simulink model "scMobileRobotLogicalArchitecture_Initial"  (R2022a)
settings: Solver=VariableStepAuto  StartTime=0.0  StopTime=10.0  RelTol=1e-3
model workspace (MAT data in the model file):
  CameraInterface = Simulink.Bus
  CameraInterface.Alignment = -1
  CameraInterface.PreserveElementDimensions = 0
  CameraInterface.Elements_internal(1) = Simulink.BusElement
  CameraInterface.Elements_internal(1).DimensionsMode = 'Fixed'
  CameraInterface.Elements_internal(1).SamplingMode = 'Sample based'
  CameraInterface.Elements_internal(1).SampleTime = -1
  CameraInterface.Elements_internal(1).Name = 'imageData'
  CameraInterface.Elements_internal(1).DataType_internal = 'uint16'
  CameraInterface.Elements_internal(1).Complexity = 'real'
  CameraInterface.Elements_internal(1).Dimensions = 1
  CameraInterface.Elements_internal(2) = Simulink.BusElement
  CameraInterface.Elements_internal(2).DimensionsMode = 'Fixed'
  CameraInterface.Elements_internal(2).SamplingMode = 'Sample based'
  CameraInterface.Elements_internal(2).SampleTime = -1
  CameraInterface.Elements_internal(2).Name = 'geoLoc'
  CameraInterface.Elements_internal(2).DataType_internal = 'double'
  CameraInterface.Elements_internal(2).Complexity = 'real'
  CameraInterface.Elements_internal(2).Dimensions = 1
  CameraInterface.Elements_internal(3) = Simulink.BusElement
  CameraInterface.Elements_internal(3).DimensionsMode = 'Fixed'
  CameraInterface.Elements_internal(3).SamplingMode = 'Sample based'
  CameraInterface.Elements_internal(3).SampleTime = -1
  CameraInterface.Elements_internal(3).Name = 'healthCheck'
  CameraInterface.Elements_internal(3).DataType_internal = 'int8'
  CameraInterface.Elements_internal(3).Complexity = 'real'
  CameraInterface.Elements_internal(3).Dimensions = 1
  CameraInterface.DataScope = 'Auto'
  CommandType = Simulink.ValueType
  CommandType.DataType = 'Enum: CommandEnum'
  GroundInterface = Simulink.ConnectionBus
  GroundInterface.Elements_internal(1) = Simulink.ConnectionElement
  GroundInterface.Elements_internal(1).Name = 'fixture'
  GroundInterface.Elements_internal(1).Type_internal = 'foundation.mechanical.translational.translational'
  GroundInterface.Elements_internal(2) = Simulink.ConnectionElement
  GroundInterface.Elements_internal(2).Name = 'socket'
  GroundInterface.Elements_internal(2).Type_internal = 'foundation.mechanical.rotational.rotational'
settings Model: Creator=The MathWorks, Inc.  LastModifiedBy=The MathWorks, Inc.
settings SolverCC: AlgebraicLoopSolver=TrustRegion  AutoInsertRateTranBlk=on  MaxZcPerStep=1
settings DebuggingCC: UnconnectedInputMsg=warning  UnconnectedOutputMsg=warning  UnconnectedLineMsg=warning  SFMachineParentedDataDiag=warning
settings ModelReferenceCC: ModelReferenceNumInstancesAllowed=Single
settings RTWCC: DLArmComputeVersion=19.05

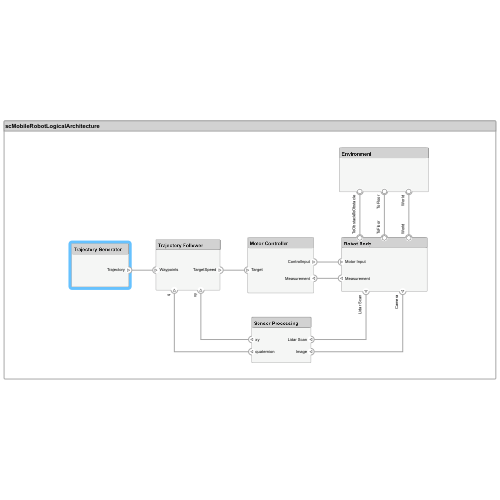
[thumbnail: Simulink's stored preview of the top-level diagram]
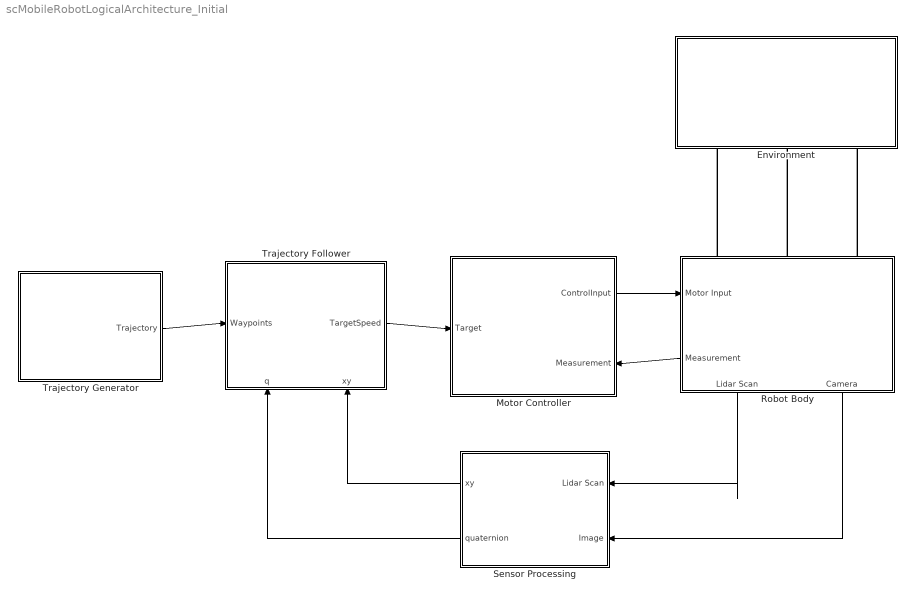
== system scMobileRobotLogicalArchitecture_Initial ==
  Environment : Subsystem
      settings: PortSchema="{\"entries\":[{\"content\":{\"headerSize\":26,\"margin\":15,\"minimumSpacing\":25,\"sides\":[{\"content\":{\"connectorIds\":[]},\"type\":\"ConnectorPlacement.EquallySpacedRectSide\",\"uuid\":\"636813ac-2488-43df-bc25-3d2ab9c69d6b\"},{\"content\":{\"connectorIds\":[],\"side\":\"RIGHT\"},\"type\":\"ConnectorPlacement.EquallySpacedRectSide\",\"uuid\":\"1c2f400a-ff06-4f0e-a520-9265bac3a8ff\"},{\"content\":{\"connectorIds\":[],\"side\":\"TOP\"},\"type\":\"ConnectorPlacement.EquallySpacedRectSide\",\"uuid\":\"d5f4b502-bbaf-4090-8459-ed02c902b998\"},{\"content\":{\"connectorIds\":[\"RConn3\",\"RConn2\",\"RConn1\"],\"side\":\"BOTTOM\"},\"type\":\"ConnectorPlacement.EquallySpacedRectSide\",\"uuid\":\"3c671e67-af17-451c-8a34-1dfdb4b38d1c\"}]},\"type\":\"ConnectorPlacement.EquallySpacedConnector\",\"uuid\":\"3f52239f-e2f4-4f3e-8b4f-59ce64028ef0\"}],\"packageUris\":[\"http://schema.mathworks.com/mf0/Connector/R2020b\"],\"version\":\"1.0\"}"
  Motor Controller : Subsystem
      settings: PortSchema="{\"entries\":[{\"content\":{\"headerSize\":26,\"margin\":15,\"minimumSpacing\":25,\"sides\":[{\"content\":{\"connectorIds\":[\"In1\"]},\"type\":\"ConnectorPlacement.EquallySpacedRectSide\",\"uuid\":\"dd0e636b-33e2-4466-b9cb-8a0d664049c0\"},{\"content\":{\"connectorIds\":[\"Out1\",\"In2\"],\"side\":\"RIGHT\"},\"type\":\"ConnectorPlacement.EquallySpacedRectSide\",\"uuid\":\"dcc76af8-d318-4ee1-8ad7-f8b5e8f6c9bf\"},{\"content\":{\"connectorIds\":[],\"side\":\"TOP\"},\"type\":\"ConnectorPlacement.EquallySpacedRectSide\",\"uuid\":\"6f591897-52d2-46bf-92a3-63841e00c811\"}]},\"type\":\"ConnectorPlacement.EquallySpacedConnector\",\"uuid\":\"27a1f739-9693-4a32-826a-45a19a2dac76\"}],\"packageUris\":[\"http://schema.mathworks.com/mf0/Connector/R2020b\"],\"version\":\"1.0\"}"
  Robot Body : Subsystem
      settings: PortSchema="{\"entries\":[{\"content\":{\"headerSize\":26,\"margin\":15,\"minimumSpacing\":25,\"sides\":[{\"content\":{\"connectorIds\":[\"In1\",\"Out3\"]},\"type\":\"ConnectorPlacement.EquallySpacedRectSide\",\"uuid\":\"636813ac-2488-43df-bc25-3d2ab9c69d6b\"},{\"content\":{\"connectorIds\":[],\"side\":\"RIGHT\"},\"type\":\"ConnectorPlacement.EquallySpacedRectSide\",\"uuid\":\"1c2f400a-ff06-4f0e-a520-9265bac3a8ff\"},{\"content\":{\"connectorIds\":[\"LConn3\",\"LConn2\",\"LConn1\"],\"side\":\"TOP\"},\"type\":\"ConnectorPlacement.EquallySpacedRectSide\",\"uuid\":\"d5f4b502-bbaf-4090-8459-ed02c902b998\"},{\"content\":{\"connectorIds\":[\"Out1\",\"Out2\"],\"side\":\"BOTTOM\"},\"type\":\"ConnectorPlacement.EquallySpacedRectSide\",\"uuid\":\"00a6c3b0-4ef2-41fb-b5f8-387f8cf4f6d5\"}]},\"type\":\"ConnectorPlacement.EquallySpacedConnector\",\"uuid\":\"3f52239f-e2f4-4f3e-8b4f-59ce64028ef0\"}],\"packageUris\":[\"http://schema.mathworks.com/mf0/Connector/R2020b\"],\"version\":\"1.0\"}"
  Sensor Processing : Subsystem
      settings: PortSchema="{\"entries\":[{\"content\":{\"headerSize\":26,\"margin\":15,\"minimumSpacing\":25,\"sides\":[{\"content\":{\"connectorIds\":[\"Out1\",\"Out2\"]},\"type\":\"ConnectorPlacement.EquallySpacedRectSide\",\"uuid\":\"85f56e06-ca1f-4c96-8cca-12b6bc6267a4\"},{\"content\":{\"connectorIds\":[\"In1\",\"In2\"],\"side\":\"RIGHT\"},\"type\":\"ConnectorPlacement.EquallySpacedRectSide\",\"uuid\":\"9cc94d56-a800-4d28-b2d9-4674df5d80f8\"},{\"content\":{\"connectorIds\":[],\"side\":\"TOP\"},\"type\":\"ConnectorPlacement.EquallySpacedRectSide\",\"uuid\":\"1ff7386a-cfbc-4c27-91ef-18689b64a000\"}]},\"type\":\"ConnectorPlacement.EquallySpacedConnector\",\"uuid\":\"4ebe64fe-780b-4293-881f-f2885e0ec8a5\"}],\"packageUris\":[\"http://schema.mathworks.com/mf0/Connector/R2020b\"],\"version\":\"1.0\"}"
  Trajectory Follower : Subsystem
      settings: PortSchema="{\"entries\":[{\"content\":{\"headerSize\":26,\"margin\":15,\"minimumSpacing\":25,\"sides\":[{\"content\":{\"connectorIds\":[\"In1\"]},\"type\":\"ConnectorPlacement.EquallySpacedRectSide\",\"uuid\":\"dd0e636b-33e2-4466-b9cb-8a0d664049c0\"},{\"content\":{\"connectorIds\":[\"Out1\"],\"side\":\"RIGHT\"},\"type\":\"ConnectorPlacement.EquallySpacedRectSide\",\"uuid\":\"dcc76af8-d318-4ee1-8ad7-f8b5e8f6c9bf\"},{\"content\":{\"connectorIds\":[],\"side\":\"TOP\"},\"type\":\"ConnectorPlacement.EquallySpacedRectSide\",\"uuid\":\"6f591897-52d2-46bf-92a3-63841e00c811\"},{\"content\":{\"connectorIds\":[\"In3\",\"In2\"],\"side\":\"BOTTOM\"},\"type\":\"ConnectorPlacement.EquallySpacedRectSide\",\"uuid\":\"93bb2a31-952b-41c1-9b16-95f23bebe0f8\"}]},\"type\":\"ConnectorPlacement.EquallySpacedConnector\",\"uuid\":\"27a1f739-9693-4a32-826a-45a19a2dac76\"}],\"packageUris\":[\"http://schema.mathworks.com/mf0/Connector/R2020b\"],\"version\":\"1.0\"}"
  Trajectory Generator : Subsystem
      settings: PortSchema="{\"entries\":[{\"content\":{\"headerSize\":26,\"margin\":15,\"minimumSpacing\":25,\"sides\":[{\"content\":{\"connectorIds\":[]},\"type\":\"ConnectorPlacement.EquallySpacedRectSide\",\"uuid\":\"dd0e636b-33e2-4466-b9cb-8a0d664049c0\"},{\"content\":{\"connectorIds\":[\"Out1\"],\"side\":\"RIGHT\"},\"type\":\"ConnectorPlacement.EquallySpacedRectSide\",\"uuid\":\"dcc76af8-d318-4ee1-8ad7-f8b5e8f6c9bf\"},{\"content\":{\"connectorIds\":[],\"side\":\"TOP\"},\"type\":\"ConnectorPlacement.EquallySpacedRectSide\",\"uuid\":\"6f591897-52d2-46bf-92a3-63841e00c811\"}]},\"type\":\"ConnectorPlacement.EquallySpacedConnector\",\"uuid\":\"27a1f739-9693-4a32-826a-45a19a2dac76\"}],\"packageUris\":[\"http://schema.mathworks.com/mf0/Connector/R2020b\"],\"version\":\"1.0\"}"
  wires:
  Sensor Processing/2(quaternion) -> Trajectory Follower/3(q)
  Sensor Processing/1(xy) -> Trajectory Follower/2(xy)
  Trajectory Follower/1(TargetSpeed) -> Motor Controller/1(Target)
  Trajectory Generator/1(Trajectory) -> Trajectory Follower/1(Waypoints)
  Motor Controller/1(ControlInput) -> Robot Body/1(Motor Input)
  Robot Body/3(Measurement) -> Motor Controller/2(Measurement)
  Robot Body/1(Lidar Scan) -> Sensor Processing/1(Lidar Scan)
  Robot Body/2(Camera) -> Sensor Processing/2(Image)
  connections:
  Robot Body/LConn2 -- Environment/RConn2
  Robot Body/LConn3 -- Environment/RConn3
  Robot Body/LConn1 -- Environment/RConn1

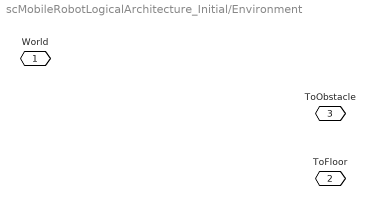
== system scMobileRobotLogicalArchitecture_Initial/Environment ==
  World : PMIOPort  Side=Right
  ToFloor : PMIOPort  Port=2  Side=Right
  ToObstacle : PMIOPort  Port=3  Side=Right

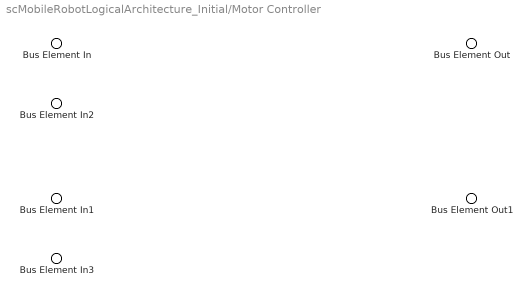
== system scMobileRobotLogicalArchitecture_Initial/Motor Controller ==
  Bus Element In1 : Inport  PortName=Target  Element=Wheel2
  Bus Element In : Inport  PortName=Target  Element=Wheel1
  Bus Element In3 : Inport  Port=2  PortName=Measurement  Element=Wheel2
  Bus Element In2 : Inport  Port=2  PortName=Measurement  Element=Wheel1
  Bus Element Out : Outport  PortName=ControlInput  Element=signal1
  Bus Element Out1 : Outport  PortName=ControlInput  Element=signal2

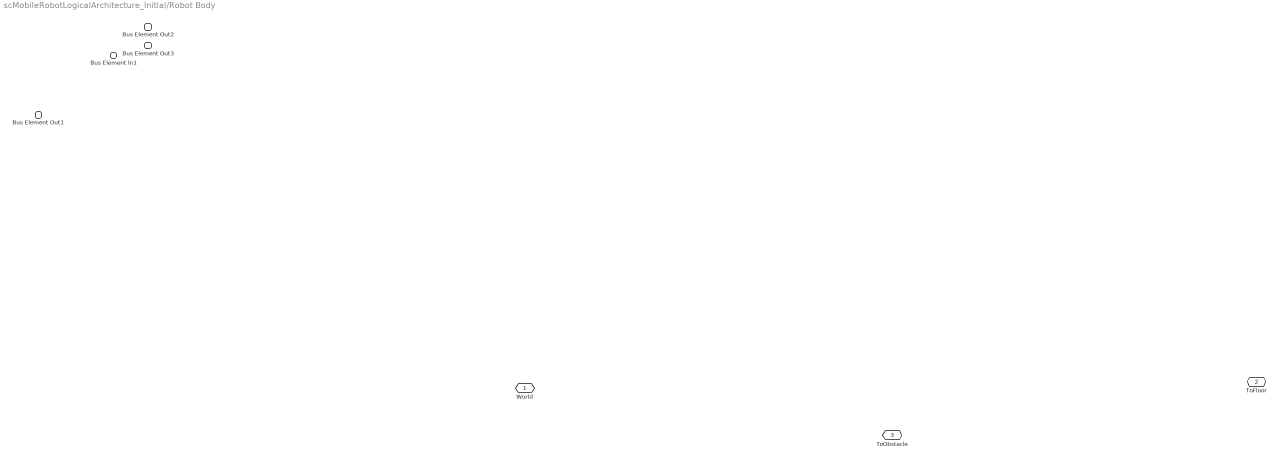
== system scMobileRobotLogicalArchitecture_Initial/Robot Body ==
  Bus Element In1 : Inport  PortName=Motor Input
  World : PMIOPort  Side=Left
  ToFloor : PMIOPort  Port=2  Side=Left
  ToObstacle : PMIOPort  Port=3  Side=Left
  Bus Element Out2 : Outport  PortName=Lidar Scan
  Bus Element Out3 : Outport  Port=2  PortName=Camera
  Bus Element Out1 : Outport  Port=3  PortName=Measurement

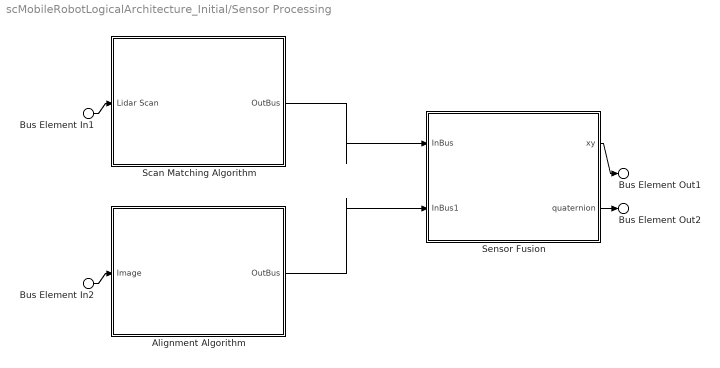
== system scMobileRobotLogicalArchitecture_Initial/Sensor Processing ==
  Bus Element In1 : Inport  PortName=Lidar Scan
  Bus Element In2 : Inport  Port=2  PortName=Image
  Alignment Algorithm : Subsystem
      settings: PortSchema="{\"entries\":[{\"content\":{\"headerSize\":26,\"margin\":15,\"minimumSpacing\":25,\"sides\":[{\"content\":{\"connectorIds\":[\"In1\"]},\"type\":\"ConnectorPlacement.EquallySpacedRectSide\",\"uuid\":\"85f56e06-ca1f-4c96-8cca-12b6bc6267a4\"},{\"content\":{\"connectorIds\":[\"Out1\"],\"side\":\"RIGHT\"},\"type\":\"ConnectorPlacement.EquallySpacedRectSide\",\"uuid\":\"9cc94d56-a800-4d28-b2d9-4674df5d80f8\"},{\"content\":{\"connectorIds\":[],\"side\":\"TOP\"},\"type\":\"ConnectorPlacement.EquallySpacedRectSide\",\"uuid\":\"1ff7386a-cfbc-4c27-91ef-18689b64a000\"}]},\"type\":\"ConnectorPlacement.EquallySpacedConnector\",\"uuid\":\"4ebe64fe-780b-4293-881f-f2885e0ec8a5\"}],\"packageUris\":[\"http://schema.mathworks.com/mf0/Connector/R2020b\"],\"version\":\"1.0\"}"
  Scan Matching Algorithm : Subsystem
      settings: PortSchema="{\"entries\":[{\"content\":{\"headerSize\":26,\"margin\":15,\"minimumSpacing\":25,\"sides\":[{\"content\":{\"connectorIds\":[\"In1\"]},\"type\":\"ConnectorPlacement.EquallySpacedRectSide\",\"uuid\":\"85f56e06-ca1f-4c96-8cca-12b6bc6267a4\"},{\"content\":{\"connectorIds\":[\"Out1\"],\"side\":\"RIGHT\"},\"type\":\"ConnectorPlacement.EquallySpacedRectSide\",\"uuid\":\"9cc94d56-a800-4d28-b2d9-4674df5d80f8\"},{\"content\":{\"connectorIds\":[],\"side\":\"TOP\"},\"type\":\"ConnectorPlacement.EquallySpacedRectSide\",\"uuid\":\"1ff7386a-cfbc-4c27-91ef-18689b64a000\"}]},\"type\":\"ConnectorPlacement.EquallySpacedConnector\",\"uuid\":\"4ebe64fe-780b-4293-881f-f2885e0ec8a5\"}],\"packageUris\":[\"http://schema.mathworks.com/mf0/Connector/R2020b\"],\"version\":\"1.0\"}"
  Sensor Fusion : Subsystem
      settings: PortSchema="{\"entries\":[{\"content\":{\"headerSize\":26,\"margin\":15,\"minimumSpacing\":25,\"sides\":[{\"content\":{\"connectorIds\":[\"In1\",\"In2\"]},\"type\":\"ConnectorPlacement.EquallySpacedRectSide\",\"uuid\":\"85f56e06-ca1f-4c96-8cca-12b6bc6267a4\"},{\"content\":{\"connectorIds\":[\"Out1\",\"Out2\"],\"side\":\"RIGHT\"},\"type\":\"ConnectorPlacement.EquallySpacedRectSide\",\"uuid\":\"9cc94d56-a800-4d28-b2d9-4674df5d80f8\"},{\"content\":{\"connectorIds\":[],\"side\":\"TOP\"},\"type\":\"ConnectorPlacement.EquallySpacedRectSide\",\"uuid\":\"1ff7386a-cfbc-4c27-91ef-18689b64a000\"}]},\"type\":\"ConnectorPlacement.EquallySpacedConnector\",\"uuid\":\"4ebe64fe-780b-4293-881f-f2885e0ec8a5\"}],\"packageUris\":[\"http://schema.mathworks.com/mf0/Connector/R2020b\"],\"version\":\"1.0\"}"
  Bus Element Out1 : Outport  PortName=xy
  Bus Element Out2 : Outport  Port=2  PortName=quaternion
  wires:
  Bus Element In1/1 -> Scan Matching Algorithm/1(Lidar Scan)
  Bus Element In2/1 -> Alignment Algorithm/1(Image)
  Scan Matching Algorithm/1(OutBus) -> Sensor Fusion/1(InBus)
  Alignment Algorithm/1(OutBus) -> Sensor Fusion/2(InBus1)
  Sensor Fusion/2(quaternion) -> Bus Element Out2/1
  Sensor Fusion/1(xy) -> Bus Element Out1/1

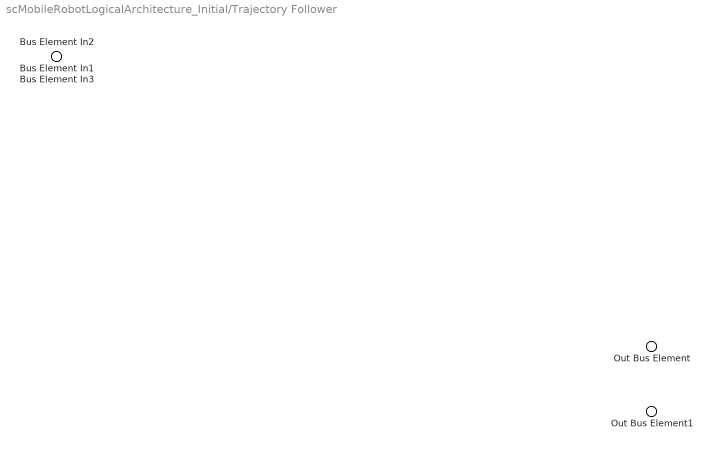
== system scMobileRobotLogicalArchitecture_Initial/Trajectory Follower ==
  Bus Element In1 : Inport  PortName=Waypoints
  Bus Element In2 : Inport  Port=2  PortName=xy
  Bus Element In3 : Inport  Port=3  PortName=q
  Out Bus Element : Outport  PortName=TargetSpeed  Element=Wheel1
  Out Bus Element1 : Outport  PortName=TargetSpeed  Element=Wheel2

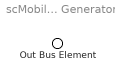
== system scMobileRobotLogicalArchitecture_Initial/Trajectory Generator ==
  Out Bus Element : Outport  PortName=Trajectory

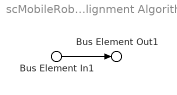
== system scMobileRobotLogicalArchitecture_Initial/Sensor Processing/Alignment Algorithm ==
  Bus Element In1 : Inport  PortName=Image
  Bus Element Out1 : Outport  PortName=OutBus
  wires:
  Bus Element In1/1 -> Bus Element Out1/1

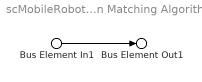
== system scMobileRobotLogicalArchitecture_Initial/Sensor Processing/Scan Matching Algorithm ==
  Bus Element In1 : Inport  PortName=Lidar Scan
  Bus Element Out1 : Outport  PortName=OutBus
  wires:
  Bus Element In1/1 -> Bus Element Out1/1

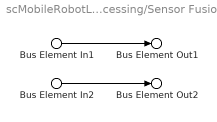
== system scMobileRobotLogicalArchitecture_Initial/Sensor Processing/Sensor Fusion ==
  Bus Element In1 : Inport  PortName=InBus
  Bus Element In2 : Inport  Port=2  PortName=InBus1
  Bus Element Out1 : Outport  PortName=xy
  Bus Element Out2 : Outport  Port=2  PortName=quaternion
  wires:
  Bus Element In1/1 -> Bus Element Out1/1
  Bus Element In2/1 -> Bus Element Out2/1
